simulink model "groundContact"  (R2024a)
settings: configuration reference "standardSILConfiguraitonParams" (kept outside this file)
libraries: matrix_library x3, simulink x1
settings Model: Creator=GTAR  LastModifiedBy=jerem
settings ConfigSetRef: SourceName=standardSILConfiguraitonParams  SourceLocation=Base Workspace

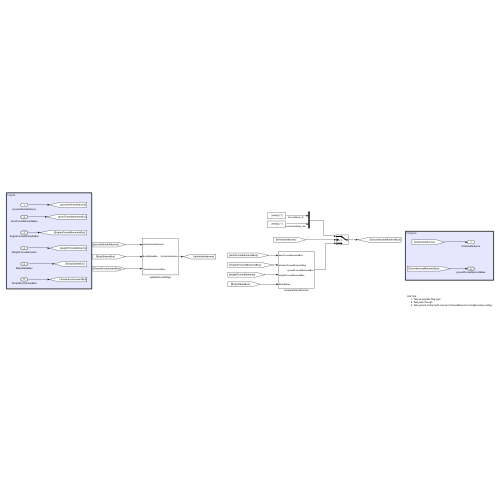
[thumbnail: Simulink's stored preview of the top-level diagram]
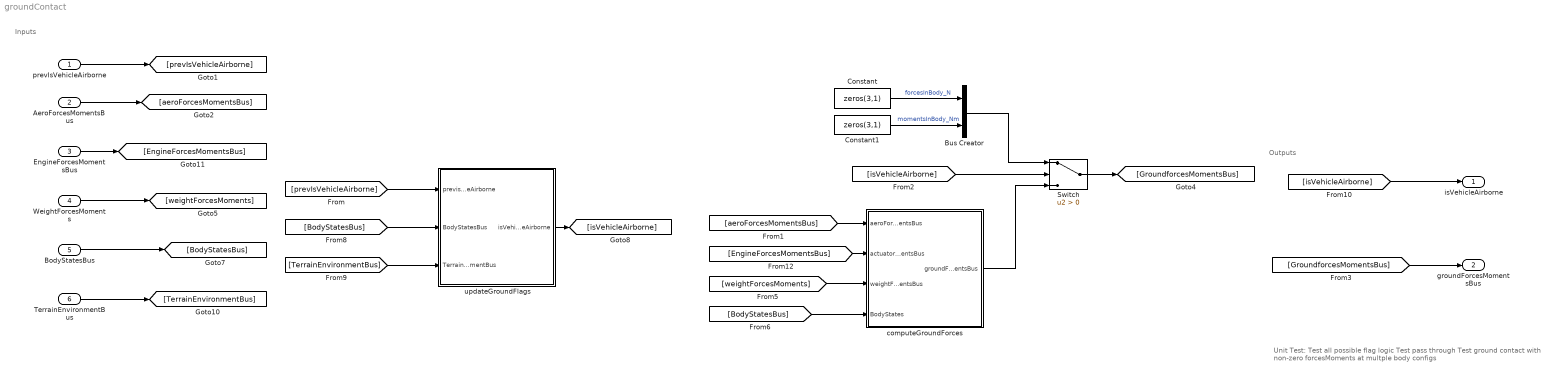
== system groundContact ==
  note: Unit Test:
      | Test all possible flag logic
      | Test pass through
      | Test ground contact with non-zero forcesMoments at multple body configs
  note: Outputs
  note: Inputs
  prevIsVehicleAirborne : Inport  OutDataTypeStr=boolean
  AeroForcesMomentsBus : Inport  Port=2  OutDataTypeStr=Bus: ComponentForcesMomentsBus
  EngineForcesMomentsBus : Inport  Port=3  OutDataTypeStr=Bus: ComponentForcesMomentsBus
  WeightForcesMoments : Inport  Port=4  OutDataTypeStr=Bus: ComponentForcesMomentsBus
  BodyStatesBus : Inport  Port=5  OutDataTypeStr=Bus: BodyStateBus
  TerrainEnvironmentBus : Inport  Port=6  OutDataTypeStr=Bus: TerrainEnvironmentBus
  Bus Creator : BusCreator  Inputs=2  OutDataTypeStr=Bus: ComponentForcesMomentsBus
  Constant : Constant  Value=zeros(3,1)
  Constant1 : Constant  Value=zeros(3,1)
  Switch : Switch  Criteria=u2 > Threshold  SaturateOnIntegerOverflow=off  InputSameDT=off
  computeGroundForces : Subsystem
  updateGroundFlags : Subsystem
  isVehicleAirborne : Outport  OutDataTypeStr=boolean
  groundForcesMomentsBus : Outport  Port=2  OutDataTypeStr=Bus: ComponentForcesMomentsBus
  wires:
  AeroForcesMomentsBus/1 -> [aeroForcesMomentsBus]
  prevIsVehicleAirborne/1 -> [prevIsVehicleAirborne]
  [prevIsVehicleAirborne] -> updateGroundFlags/1(previsVehicleAirborne)
  [isVehicleAirborne] -> Switch/2
  WeightForcesMoments/1 -> [weightForcesMoments]
  BodyStatesBus/1 -> [BodyStatesBus]
  [GroundforcesMomentsBus] -> groundForcesMomentsBus/1
  [BodyStatesBus] -> updateGroundFlags/2(BodyStatesBus)
  [TerrainEnvironmentBus] -> updateGroundFlags/3(TerrainEnvironmentBus)
  updateGroundFlags/1(isVehicleAirborne) -> [isVehicleAirborne]
  [isVehicleAirborne] -> isVehicleAirborne/1
  TerrainEnvironmentBus/1 -> [TerrainEnvironmentBus]
  EngineForcesMomentsBus/1 -> [EngineForcesMomentsBus]
  [aeroForcesMomentsBus] -> computeGroundForces/1(aeroForcesMomentsBus)
  [EngineForcesMomentsBus] -> computeGroundForces/2(actuatorForcesMomentsBus)
  [weightForcesMoments] -> computeGroundForces/3(weightForcesMomentsBus)
  [BodyStatesBus] -> computeGroundForces/4(BodyStates)
  Constant/1 -> Bus Creator/1  "forcesInBody_N"
  Constant1/1 -> Bus Creator/2  "momentsInBody_Nm"
  computeGroundForces/1(groundForcesMomentsBus) -> Switch/3
  Switch/1 -> [GroundforcesMomentsBus]
  Bus Creator/1 -> Switch/1

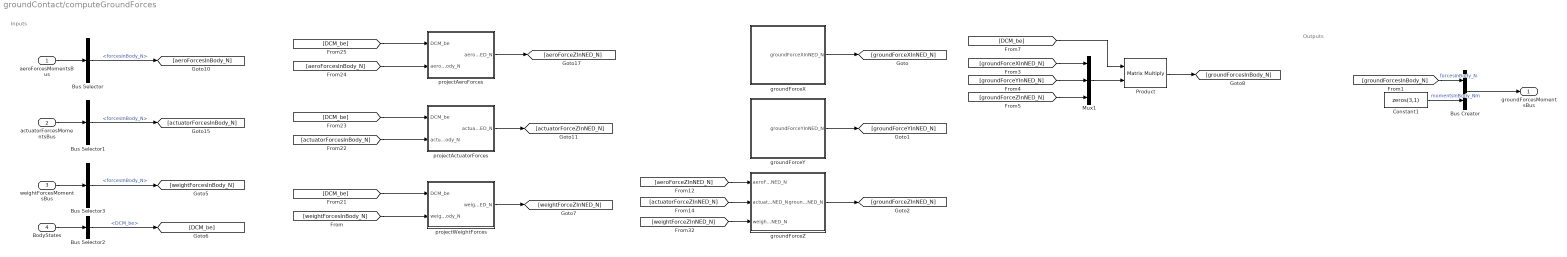
== system groundContact/computeGroundForces ==
  note: Inputs
  note: Outputs
  aeroForcesMomentsBus : Inport  OutDataTypeStr=Bus: ComponentForcesMomentsBus
  actuatorForcesMomentsBus : Inport  Port=2  OutDataTypeStr=Bus: ComponentForcesMomentsBus
  weightForcesMomentsBus : Inport  Port=3  OutDataTypeStr=Bus: ComponentForcesMomentsBus
  BodyStates : Inport  Port=4  OutDataTypeStr=Bus: BodyStateBus
  Bus Creator : BusCreator  Inputs=2  OutDataTypeStr=Bus: ComponentForcesMomentsBus
  Bus Selector : BusSelector  OutputSignals=forcesInBody_N
  Bus Selector1 : BusSelector  OutputSignals=forcesInBody_N
  Bus Selector2 : BusSelector  OutputSignals=DCM_be
  Bus Selector3 : BusSelector  OutputSignals=forcesInBody_N
  Constant1 : Constant  Value=zeros(3,1)
  Mux1 : Mux  Inputs=3
  Product : Product  Multiplication=Matrix(*)
  groundForceX : Subsystem
  groundForceY : Subsystem
  groundForceZ : Subsystem
  projectActuatorForces : Subsystem
  projectAeroForces : Subsystem
  projectWeightForces : Subsystem
  groundForcesMomentsBus : Outport  OutDataTypeStr=Bus: ComponentForcesMomentsBus
  wires:
  aeroForcesMomentsBus/1 -> Bus Selector/1
  groundForceX/1(groundForceXInNED_N) -> [groundForceXInNED_N]
  groundForceY/1(groundForceYInNED_N) -> [groundForceYInNED_N]
  groundForceZ/1(groundForceZInNED_N) -> [groundForceZInNED_N]
  [aeroForceZInNED_N] -> groundForceZ/1(aeroForceZInNED_N)
  [actuatorForceZInNED_N] -> groundForceZ/2(actuatorForceZInNED_N)
  [groundForceXInNED_N] -> Mux1/1
  [groundForceYInNED_N] -> Mux1/2
  [groundForceZInNED_N] -> Mux1/3
  Mux1/1 -> Product/2
  [DCM_be] -> Product/1
  actuatorForcesMomentsBus/1 -> Bus Selector1/1
  Bus Selector/1 -> [aeroForcesInBody_N]  "<forcesInBody_N>"
  BodyStates/1 -> Bus Selector2/1
  Bus Selector2/1 -> [DCM_be]  "<DCM_be>"
  [groundForcesInBody_N] -> Bus Creator/1  "forcesInBody_N"
  Product/1 -> [groundForcesInBody_N]
  weightForcesMomentsBus/1 -> Bus Selector3/1
  Bus Selector3/1 -> [weightForcesInBody_N]  "<forcesInBody_N>"
  [DCM_be] -> projectWeightForces/1(DCM_be)
  [weightForcesInBody_N] -> projectWeightForces/2(weightForcesInBody_N)
  projectWeightForces/1(weightForceZInNED_N) -> [weightForceZInNED_N]
  projectActuatorForces/1(actuatorForceZInNED_N) -> [actuatorForceZInNED_N]
  [actuatorForcesInBody_N] -> projectActuatorForces/2(actuatorForcesInBody_N)
  [DCM_be] -> projectActuatorForces/1(DCM_be)
  [DCM_be] -> projectAeroForces/1(DCM_be)
  [aeroForcesInBody_N] -> projectAeroForces/2(aeroForcesInBody_N)
  projectAeroForces/1(aeroForceZInNED_N) -> [aeroForceZInNED_N]
  Bus Selector1/1 -> [actuatorForcesInBody_N]  "<forcesInBody_N>"
  [weightForceZInNED_N] -> groundForceZ/3(weightForceZInNED_N)
  Bus Creator/1 -> groundForcesMomentsBus/1
  Constant1/1 -> Bus Creator/2  "momentsInBody_Nm"

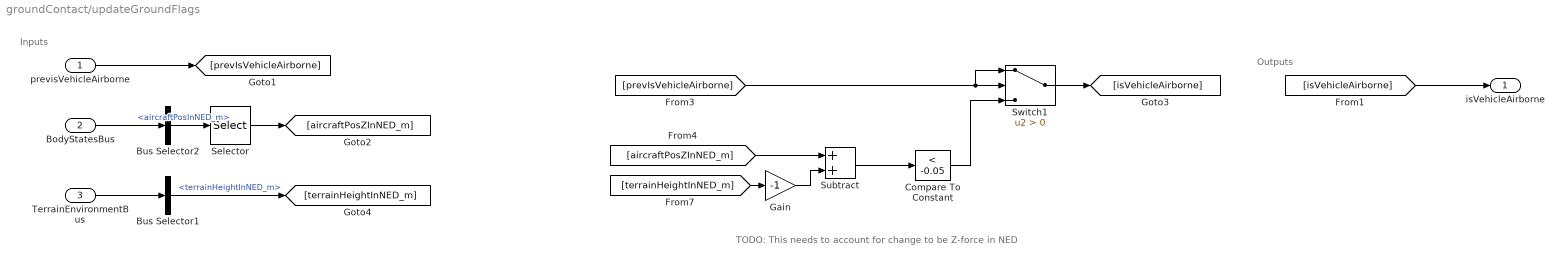
== system groundContact/updateGroundFlags ==
  note: TODO: This needs to account for change to be Z-force in NED
  note: Outputs
  note: Inputs
  previsVehicleAirborne : Inport  OutDataTypeStr=boolean
  BodyStatesBus : Inport  Port=2  OutDataTypeStr=Bus: BodyStateBus
  TerrainEnvironmentBus : Inport  Port=3  OutDataTypeStr=Bus: TerrainEnvironmentBus
  Bus Selector1 : BusSelector  OutputSignals=terrainHeightInNED_m
  Bus Selector2 : BusSelector  OutputSignals=aircraftPosInNED_m
  Compare To Constant : simulink/Logic and Bit Operations/Compare To Constant  relop=<  const=-0.05  OutDataTypeStr=boolean
  Gain : Gain  Gain=-1
  Selector : Selector  InputPortWidth=3  IndexOptions=Index vector (dialog)  Indices=3  OutputSizes=1
  Subtract : Sum
  Switch1 : Switch  Criteria=u2 > Threshold  SaturateOnIntegerOverflow=off  InputSameDT=off
  isVehicleAirborne : Outport  OutDataTypeStr=boolean
  wires:
  TerrainEnvironmentBus/1 -> Bus Selector1/1
  previsVehicleAirborne/1 -> [prevIsVehicleAirborne]
  BodyStatesBus/1 -> Bus Selector2/1
  [prevIsVehicleAirborne] -> Switch1/1, Switch1/2
  Switch1/1 -> [isVehicleAirborne]
  Selector/1 -> [aircraftPosZInNED_m]
  [isVehicleAirborne] -> isVehicleAirborne/1
  Bus Selector1/1 -> [terrainHeightInNED_m]  "<terrainHeightInNED_m>"
  Compare To Constant/1 -> Switch1/3
  [aircraftPosZInNED_m] -> Subtract/1
  [terrainHeightInNED_m] -> Gain/1
  Subtract/1 -> Compare To Constant/1
  Gain/1 -> Subtract/2
  Bus Selector2/1 -> Selector/1  "<aircraftPosInNED_m>"

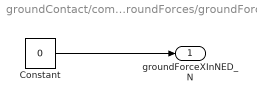
== system groundContact/computeGroundForces/groundForceX ==
  Constant : Constant  Value=0
  groundForceXInNED_N : Outport
  wires:
  Constant/1 -> groundForceXInNED_N/1

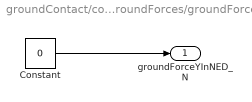
== system groundContact/computeGroundForces/groundForceY ==
  Constant : Constant  Value=0
  groundForceYInNED_N : Outport
  wires:
  Constant/1 -> groundForceYInNED_N/1

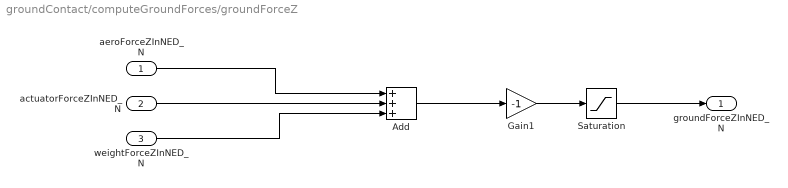
== system groundContact/computeGroundForces/groundForceZ ==
  aeroForceZInNED_N : Inport
  actuatorForceZInNED_N : Inport  Port=2
  weightForceZInNED_N : Inport  Port=3
  Add : Sum  Inputs=+++
  Gain1 : Gain  Gain=-1
  Saturation : Saturate  UpperLimit=0  LowerLimit=-inf
  groundForceZInNED_N : Outport
  wires:
  Add/1 -> Gain1/1
  aeroForceZInNED_N/1 -> Add/1
  actuatorForceZInNED_N/1 -> Add/2
  Gain1/1 -> Saturation/1
  weightForceZInNED_N/1 -> Add/3
  Saturation/1 -> groundForceZInNED_N/1

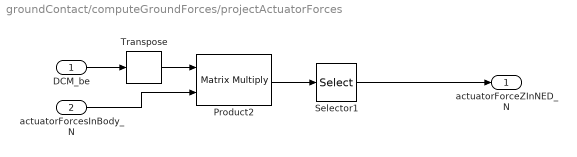
== system groundContact/computeGroundForces/projectActuatorForces ==
  DCM_be : Inport
  actuatorForcesInBody_N : Inport  Port=2
  Product2 : Product  Multiplication=Matrix(*)
  Selector1 : Selector  InputPortWidth=3  IndexOptions=Index vector (dialog)  Indices=[3]  OutputSizes=1
  Transpose : matrix_library/Transpose
  actuatorForceZInNED_N : Outport
  wires:
  actuatorForcesInBody_N/1 -> Product2/2
  Product2/1 -> Selector1/1
  Selector1/1 -> actuatorForceZInNED_N/1
  DCM_be/1 -> Transpose/1
  Transpose/1 -> Product2/1

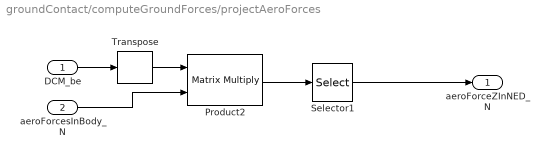
== system groundContact/computeGroundForces/projectAeroForces ==
  DCM_be : Inport
  aeroForcesInBody_N : Inport  Port=2
  Product2 : Product  Multiplication=Matrix(*)
  Selector1 : Selector  InputPortWidth=3  IndexOptions=Index vector (dialog)  Indices=[3]  OutputSizes=1
  Transpose : matrix_library/Transpose
  aeroForceZInNED_N : Outport
  wires:
  Transpose/1 -> Product2/1
  DCM_be/1 -> Transpose/1
  Selector1/1 -> aeroForceZInNED_N/1
  Product2/1 -> Selector1/1
  aeroForcesInBody_N/1 -> Product2/2

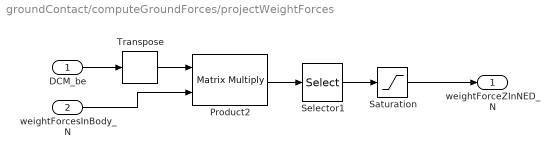
== system groundContact/computeGroundForces/projectWeightForces ==
  DCM_be : Inport
  weightForcesInBody_N : Inport  Port=2
  Product2 : Product  Multiplication=Matrix(*)
  Saturation : Saturate  UpperLimit=Inf  LowerLimit=0
  Selector1 : Selector  InputPortWidth=3  IndexOptions=Index vector (dialog)  Indices=[3]  OutputSizes=1
  Transpose : matrix_library/Transpose
  weightForceZInNED_N : Outport
  wires:
  Transpose/1 -> Product2/1
  DCM_be/1 -> Transpose/1
  Saturation/1 -> weightForceZInNED_N/1
  Product2/1 -> Selector1/1
  Selector1/1 -> Saturation/1
  weightForcesInBody_N/1 -> Product2/2
